simulink model "Laboratory_4_Problem_3_Group 5"  (R2024b)
settings: Solver=VariableStepAuto  StartTime=0.0  StopTime=Sim_Time  RelTol=1e-3
undefined symbols (not defined in the file): A, B, C, D
settings Model: Creator=User  LastModifiedBy=User

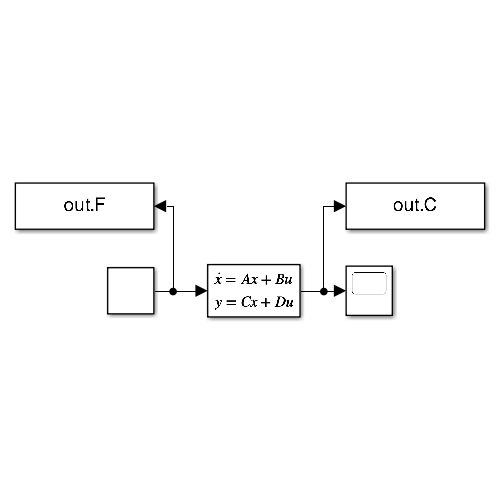
[thumbnail: Simulink's stored preview of the top-level diagram]
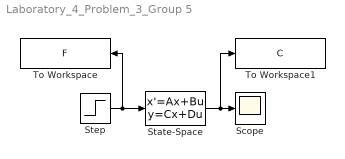
== system Laboratory_4_Problem_3_Group 5 ==
  Scope : Scope
  State-Space : StateSpace  A=A  B=B  C=C  D=D  InitialCondition=0
  Step : Step  SampleTime=0
  To Workspace : ToWorkspace  VariableName=F  SaveFormat=Timeseries  SampleTime=-1
  To Workspace1 : ToWorkspace  VariableName=C  SaveFormat=Timeseries  SampleTime=-1
  wires:
  Step/1 -> To Workspace/1, State-Space/1
  State-Space/1 -> To Workspace1/1, Scope/1
